simulink model "kalman_simulink"  (R2024a)
settings: Solver=VariableStepAuto  StartTime=0.0  StopTime=10  MaxStep=0.01  RelTol=1e-3
undefined symbols (not defined in the file): Continuous, Time
libraries: simulink x1, ctrlSharedLib x1
settings Model: Creator=SHARI  LastModifiedBy=SHARI

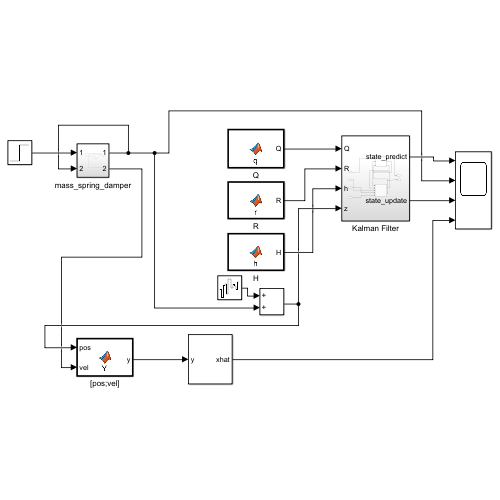
[thumbnail: Simulink's stored preview of the top-level diagram]
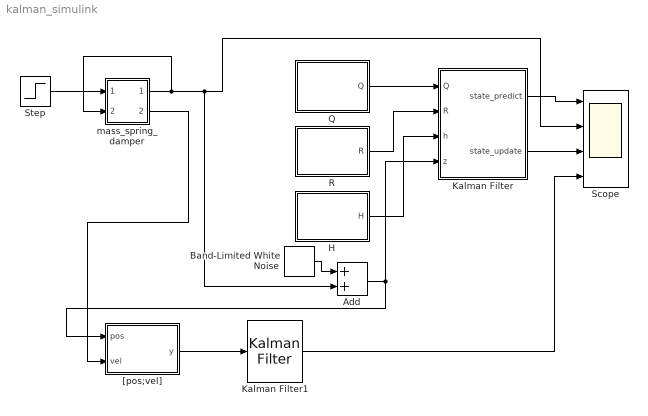
== system kalman_simulink ==
  Add : Sum
  Band-Limited White Noise : simulink/Sources/Band-Limited White Noise  Cov=[0.1]  Ts=0.1  seed=[23341]
  H : MATLAB Function  TreatAsAtomicUnit=on
  Kalman Filter : Subsystem
  Kalman Filter1 : ctrlSharedLib/Kalman Filter  TimeDomain=Continuous-Time  UseCurrentEstimator=on  ModelSource=Individual A, B, C, D matrices  ModelSourceVariable=ss(0.95,1,1,0,1)  A=[0 1; 1 1]  B=1  C=[1 0.01; 0.01 1]  D=0  NumberOfStates=1  NumberOfInputs=1  NumberOfOutputs=1  InitialEstimateSource=Dialog  X0=0  P0=10  UseK=off  UseGH=off  NumberOfProcessNoiseInputs=1  G=1  TimeInvariantG=on  H=0  TimeInvariantH=on  Q=0.05  TimeInvariantQ=on  R=1  TimeInvariantR=on  N=0  TimeInvariantN=on  AddInputPort=off  AddEnablePort=off  OutputEstimatedY=off  OutputP=off  Ts=-1
  Q : MATLAB Function  TreatAsAtomicUnit=on
  R : MATLAB Function  TreatAsAtomicUnit=on
  Scope : Scope  NumInputPorts=4
  Step : Step  SampleTime=0
  "[pos;vel]" : MATLAB Function  TreatAsAtomicUnit=on
  mass_spring_damper : Subsystem
  wires:
  Band-Limited White Noise/1 -> Add/1
  Q/1(Q) -> Kalman Filter/1(Q)
  R/1(R) -> Kalman Filter/2(R)
  H/1(H) -> Kalman Filter/3(h)
  Add/1 -> Kalman Filter/4(z), "[pos;vel]"/1(pos)
  Kalman Filter/1(state_predict) -> Scope/1
  Kalman Filter/2(state_update) -> Scope/3
  Kalman Filter1/1 -> Scope/4
  "[pos;vel]"/1(y) -> Kalman Filter1/1
  mass_spring_damper/1(Out1) -> Add/2, Scope/2, mass_spring_damper/2(In2)
  Step/1 -> mass_spring_damper/1(In1)
  mass_spring_damper/2(Out2) -> "[pos;vel]"/2(vel)

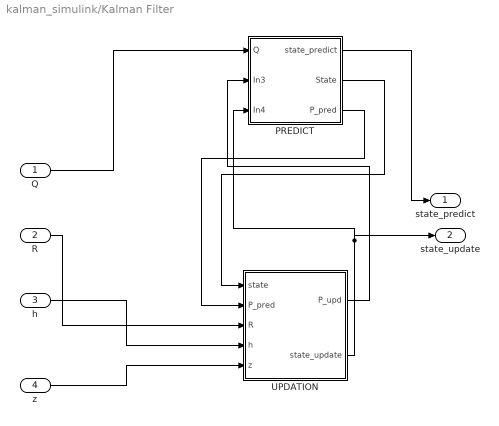
== system kalman_simulink/Kalman Filter ==
  Q : Inport
  R : Inport  Port=2
  h : Inport  Port=3
  z : Inport  Port=4
  PREDICT : Subsystem
  UPDATION : Subsystem
  state_predict : Outport
  state_update : Outport  Port=2
  wires:
  UPDATION/2(state_update) -> state_update/1, PREDICT/3(In4)
  UPDATION/1(P_upd) -> PREDICT/2(In3)
  PREDICT/2(State) -> UPDATION/1(state)
  h/1 -> UPDATION/4(h)
  PREDICT/3(P_pred) -> UPDATION/2(P_pred)
  Q/1 -> PREDICT/1(Q)
  PREDICT/1(state_predict) -> state_predict/1
  R/1 -> UPDATION/3(R)
  z/1 -> UPDATION/5(z)

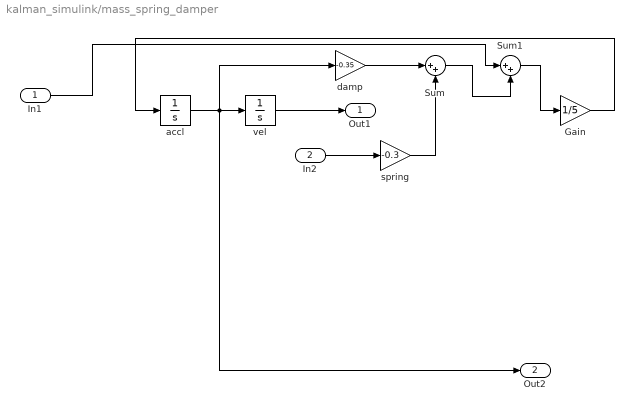
== system kalman_simulink/mass_spring_damper ==
  In1 : Inport
  In2 : Inport  Port=2
  Gain : Gain  Gain=1/5
  Sum : Sum  Inputs=|++
  Sum1 : Sum  Inputs=|++
  accl : Integrator
  damp : Gain  Gain=-0.35
  spring : Gain  Gain=-0.3
  vel : Integrator
  Out1 : Outport
  Out2 : Outport  Port=2
  wires:
  Sum/1 -> Sum1/2
  In2/1 -> spring/1
  spring/1 -> Sum/2
  vel/1 -> Out1/1
  damp/1 -> Sum/1
  accl/1 -> Out2/1, damp/1, vel/1
  In1/1 -> Sum1/1
  Sum1/1 -> Gain/1
  Gain/1 -> accl/1

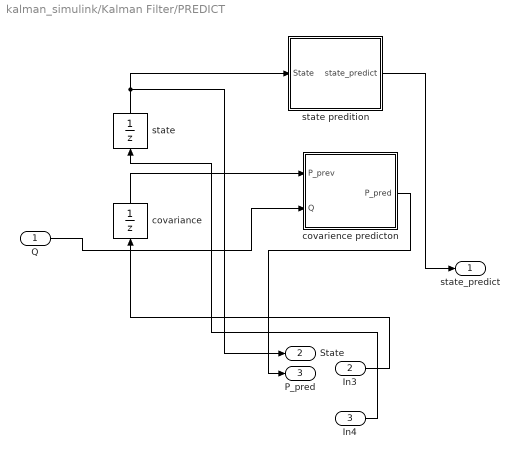
== system kalman_simulink/Kalman Filter/PREDICT ==
  Q : Inport
  In3 : Inport  Port=2
  In4 : Inport  Port=3
  " covariance" : UnitDelay  InitialCondition=[1 0.01; 0.01 1]  SampleTime=-1  HasFrameUpgradeWarning=on
  covarience predicton : MATLAB Function  TreatAsAtomicUnit=on
  state : UnitDelay  InitialCondition=[0;0]  SampleTime=-1  HasFrameUpgradeWarning=on
  "state predition " : MATLAB Function  TreatAsAtomicUnit=on
  state_predict : Outport
  State : Outport  Port=2
  P_pred : Outport  Port=3
  wires:
  state/1 -> State/1, "state predition "/1(State)
  " covariance"/1 -> covarience predicton/1(P_prev)
  "state predition "/1(state_predict) -> state_predict/1
  covarience predicton/1(P_pred) -> P_pred/1
  Q/1 -> covarience predicton/2(Q)
  In4/1 -> state/1
  In3/1 -> " covariance"/1

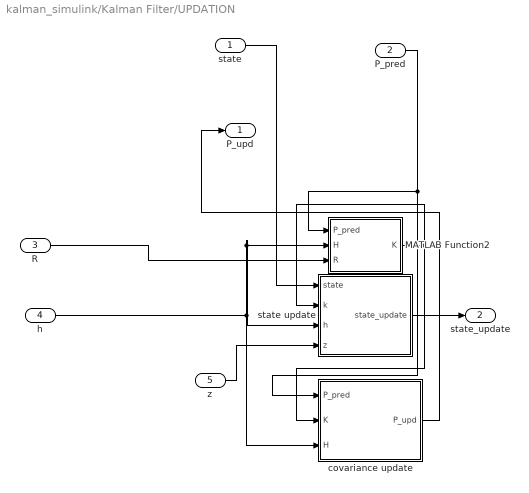
== system kalman_simulink/Kalman Filter/UPDATION ==
  state : Inport
  P_pred : Inport  Port=2
  R : Inport  Port=3
  h : Inport  Port=4
  z : Inport  Port=5
  MATLAB Function2 : MATLAB Function  TreatAsAtomicUnit=on
  covariance update : MATLAB Function  TreatAsAtomicUnit=on
  state update : MATLAB Function  TreatAsAtomicUnit=on
  P_upd : Outport
  state_update : Outport  Port=2
  wires:
  MATLAB Function2/1(K) -> state update/2(k), covariance update/2(K)
  P_pred/1 -> MATLAB Function2/1(P_pred), covariance update/1(P_pred)
  state update/1(state_update) -> state_update/1
  h/1 -> state update/3(h), MATLAB Function2/2(H), covariance update/3(H)
  covariance update/1(P_upd) -> P_upd/1
  state/1 -> state update/1(state)
  R/1 -> MATLAB Function2/3(R)
  z/1 -> state update/4(z)

== matlab function kalman_simulink/Kalman Filter/PREDICT/state predition  ==
  data: state_predict output; State input
function state_predict  = state(State)
    A = [0 1; 1 1];

    state_predict = A * State ;
end

== matlab function kalman_simulink/Kalman Filter/PREDICT/covarience predicton ==
  data: P_pred output; P_prev input; Q input
function P_pred = cov_predict( P_prev, Q)
A = [1 0.01; 0.01 1];
    P_pred = A * P_prev * A' + Q;
end

== matlab function kalman_simulink/Kalman Filter/UPDATION/state update ==
  data: state input; state_update output; k input; h input; z input
function state_update = update(state, k, h, z)
    state_update = state + k * (z - h * state);
end

== matlab function kalman_simulink/Kalman Filter/UPDATION/covariance update ==
  data: P_pred input; P_upd output; K input; H input
function P_upd = cov_update(P_pred, K, H)
    I = eye(size(P_pred));
    P_upd = (I - K * H) * P_pred;
end

== matlab function kalman_simulink/Kalman Filter/UPDATION/MATLAB Function2 ==
  data: K output; P_pred input; H input; R input
function K = gain(P_pred, H, R)
    K = P_pred * H' / (H * P_pred * H' + R);
end

== matlab function kalman_simulink/[pos;vel] ==
  data: y output; pos input; vel input
function y = Y(pos, vel)
y = [pos;vel];
end

== matlab function kalman_simulink/H ==
  data: H output
function H = h
H = [1 0]
end

== matlab function kalman_simulink/Q ==
  data: Q output
function Q  = q
Q = [0.001 0; 0 0.001];
end

== matlab function kalman_simulink/R ==
  data: R output
function R = r()
R = 0.5;
end
